simulink model "DashboardComponentsExample"  (R2022a)
settings: Solver=VariableStepAuto  StartTime=0.0  StopTime=inf  RelTol=1e-3
settings Model: Creator=bryantboatright  LastModifiedBy=boater
settings ModelReferenceCC: EnableRefExpFcnMdlSchedulingChecks=off
settings RTWCC: Description=Generic Real-Time Target

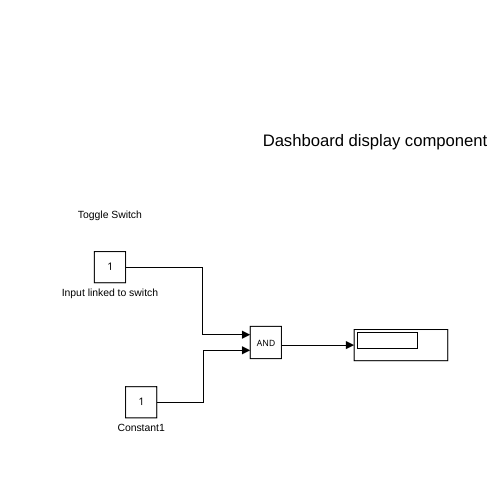
[thumbnail: Simulink's stored preview of the top-level diagram]
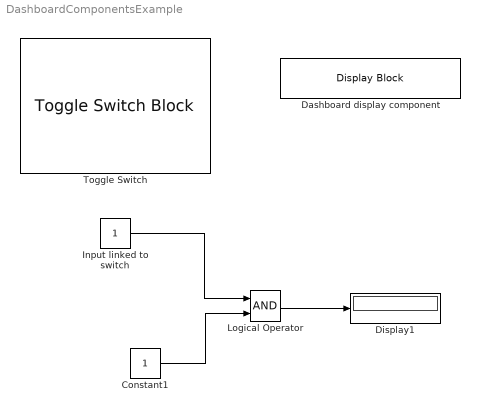
== system DashboardComponentsExample ==
  Constant1 : Constant
  Dashboard display component : DisplayBlock  LabelPosition=Hide  Transparency=1
  Display1 : Display
  Input linked to switch : Constant
  Logical Operator : Logic  AllPortsSameDT=off  OutDataTypeStr=boolean
  Toggle Switch : ToggleSwitchBlock
      settings: Values={{'Off', 'On'}, [0 1]}
  wires:
  Input linked to switch/1 -> Logical Operator/1
  Constant1/1 -> Logical Operator/2
  Logical Operator/1 -> Display1/1
